simulink model "Multiple_Monitors"  (R2015a)
settings: Solver=ode45  StartTime=0.0  StopTime=20  RelTol=1e-3
values from neighbouring files (symbols this model uses):
  Phi_1 = '[.]( p1 /\ p2) '    [Run_Demo.m]
  Phi_2 = '[.]_[0,10]( p1 /\ p2 ) '    [Run_Demo.m]
  Phi_3 = '[.]_[0,20]( !( p1 /\ p2) -> <>_[0,10] []_[0,10]( p1 /\ p2) )'    [Run_Demo.m]
  Phi_4 = '[.]( !( p1 /\ p2) -> <>_[0,10] []_[0,10]( p1 /\ p2) )'    [Run_Demo.m]
  Phi_5 = '<.>_[0,10]( p1 /\ p2) '    [Run_Demo.m]
undefined symbols (not defined in the file or in its folder): InputDimension, Preds
settings Model: Creator=adokhanc  LastModifiedBy=adokhanc

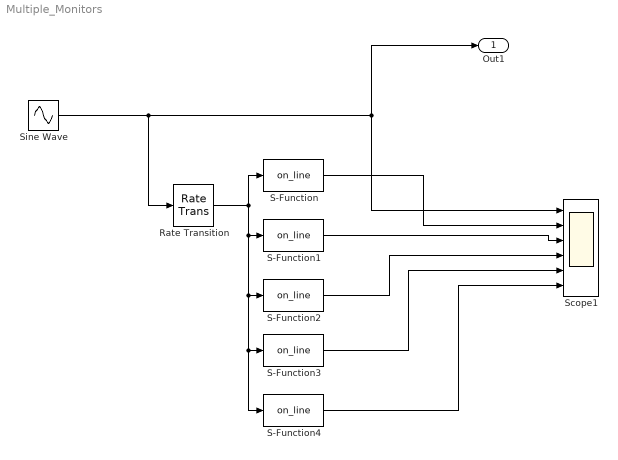
== system Multiple_Monitors ==
  Rate Transition : RateTransition  OutPortSampleTime=0.1
  S-Function : S-Function  FunctionName=on_line  Parameters=InputDimension,Phi_1,Preds
  S-Function1 : S-Function  FunctionName=on_line  Parameters=InputDimension,Phi_2,Preds
  S-Function2 : S-Function  FunctionName=on_line  Parameters=InputDimension,Phi_3,Preds
  S-Function3 : S-Function  FunctionName=on_line  Parameters=InputDimension,Phi_4,Preds
  S-Function4 : S-Function  FunctionName=on_line  Parameters=InputDimension,Phi_5,Preds
  Scope1 : Scope  NumInputPorts=6
      settings: YMin=-0~0~-5~-5~-5~-5  YMax=2~1~5~5~5~5
  Sine Wave : Sin  SampleTime=0.05
  Out1 : Outport
  wires:
  S-Function/1 -> Scope1/2
  Sine Wave/1 -> Rate Transition/1, Out1/1, Scope1/1
  S-Function1/1 -> Scope1/3
  S-Function2/1 -> Scope1/4
  S-Function3/1 -> Scope1/5
  S-Function4/1 -> Scope1/6
  Rate Transition/1 -> S-Function4/1, S-Function3/1, S-Function2/1, S-Function1/1, S-Function/1
